simulink model "sampleModel20"  (R2021a)
settings: Solver=VariableStepAuto  StartTime=0.0  StopTime=10.0  RelTol=1e-3
undefined symbols (not defined in the file): DiscIntNeverNeededParam, magnitude, Newton, Raphson
libraries: simulink x274, pid_lib x17
(part 2 of 16)

== system sampleModel20/cfblk77/cfblk9 ==
  cfblk1 : Inport
  cfblk8 : Inport  Port=2
  cfblk9 : Inport  Port=3
  cfblk10 : Inport  Port=4
  cfblk11 : Inport  Port=5
  cfblk{12..17} (6 alike) : Delay  SampleTime=1
  cfblk3 : Sin  TimeSource=Use external signal  SampleTime=0
  cfblk4 : Assignment  DiagnosticForDimensions=Warning  IndexOptions=Index vector (dialog)  Indices=1  OutputSizes=1
  cfblk5 : Subsystem
  cfblk6 : Subsystem
  cfblk7 : Subsystem
  cfblk2 : Outport
  wires:
  cfblk1/1 -> cfblk5/1(cfblk1)
  cfblk6/1(cfblk2) -> cfblk7/1(cfblk1)
  cfblk8/1 -> cfblk4/1
  cfblk9/1 -> cfblk4/2
  cfblk5/1(cfblk2) -> cfblk3/1
  cfblk11/1 -> cfblk2/1, cfblk7/4(cfblk6)
  cfblk10/1 -> cfblk5/3(cfblk8)
  cfblk4/1 -> cfblk7/2(cfblk4)
  cfblk5/2(cfblk12) -> cfblk6/2(cfblk12)
  cfblk7/2(cfblk7) -> cfblk14/1, cfblk15/1, cfblk16/1
  cfblk6/3(cfblk15) -> cfblk7/3(cfblk5)
  cfblk3/1 -> cfblk12/1
  cfblk12/1 -> cfblk5/4(cfblk9)
  cfblk7/1(cfblk2) -> cfblk13/1
  cfblk13/1 -> cfblk6/1(cfblk1)
  cfblk14/1 -> cfblk6/3(cfblk13)
  cfblk15/1 -> cfblk5/5(cfblk10)
  cfblk16/1 -> cfblk5/6(cfblk11)
  cfblk6/2(cfblk14) -> cfblk17/1
  cfblk17/1 -> cfblk5/2(cfblk7)

== system sampleModel20/cfblk78/cfblk10 ==
  cfblk1 : Inport
  cfblk9 : Inport  Port=2
  cfblk10 : Inport  Port=3
  cfblk11 : Inport  Port=4
  cfblk12 : Inport  Port=5
  cfblk{14..17} (4 alike) : Delay  SampleTime=1
  cfblk3 : pid_lib/PID Controller (2DOF)  Controller=PID  Form=Parallel  TimeDomain=Discrete-time  UseExternalTs=off  SampleTime=1  IntegratorMethod=Forward Euler  FilterMethod=Forward Euler  ControllerParametersSource=internal  P=1  I=1  D=0  UseFilter=on  N=100  b=1  c=1  TunerSelectOption=Transfer Function Based (PID Tuner App)  InitialConditionSource=internal  InitialConditionForIntegrator=0  InitialConditionForFilter=0  DifferentiatorICPrevScaledInput=0  ExternalReset=none  TrackingMode=off  Kt=1  LimitOutput=off  SatLimitsSource=internal  UpperSaturationLimit=inf  LowerSaturationLimit=-inf  LinearizeAsGain=off  AntiWindupMode=none  Kb=1  POutMin=[]  POutMax=[]  IOutMin=[]  IOutMax=[]  DOutMin=[]  DOutMax=[]  NOutMin=[]  NOutMax=[]  bOutMin=[]  bOutMax=[]  cOutMin=[]  cOutMax=[]  SumOutMin=[]  SumOutMax=[]  SaturationOutMin=[]  SaturationOutMax=[]  PParamMin=[]  PParamMax=[]  IParamMin=[]  IParamMax=[]  DParamMin=[]  DParamMax=[]  NParamMin=[]  NParamMax=[]  bParamMin=[]  bParamMax=[]  cParamMin=[]  cParamMax=[]  KbParamMin=[]  KbParamMax=[]  KtParamMin=[]  KtParamMax=[]  KbOutMin=[]  KbOutMax=[]  KtOutMin=[]  KtOutMax=[]  IntegratorOutMin=[]  IntegratorOutMax=[]  FilterOutMin=[]  FilterOutMax=[]  SumI1OutMin=[]  SumI1OutMax=[]  SumI2OutMin=[]  SumI2OutMax=[]  SumI3OutMin=[]  SumI3OutMax=[]  SumI4OutMin=[]  SumI4OutMax=[]  SumDOutMin=[]  SumDOutMax=[]  Sum1OutMin=[]  Sum1OutMax=[]  Sum2OutMin=[]  Sum2OutMax=[]  Sum3OutMin=[]  Sum3OutMax=[]  DifferentiatorOutMin=[]  DifferentiatorOutMax=[]  FilterDiffOutCoefMin=[]  FilterDiffOutCoefMax=[]  ReciprocalOutMin=[]  ReciprocalOutMax=[]  SumDenOutMin=[]  SumDenOutMax=[]  SumNumOutMin=[]  SumNumOutMax=[]  DivideOutMin=[]  DivideOutMax=[]  UdiffTsProdOutMin=[]  UdiffTsProdOutMax=[]  NTsProdOutMin=[]  NTsProdOutMax=[]  UintegralTsProdOutMin=[]  UintegralTsProdOutMax=[]  UngainTsProdOutMin=[]  UngainTsProdOutMax=[]  IntegratorContinuousStateAttributes=''  IntegratorStateMustResolveToSignalObject=off  IntegratorRTWStateStorageClass=Auto  FilterContinuousStateAttributes=''  FilterStateMustResolveToSignalObject=off  FilterRTWStateStorageClass=Auto  ParallelPVariant=InternalParameters  IdealPVariant=Disabled  IVariant=InternalParameters  DVariant=InternalParameters  bVariant=InternalParameters  cVariant=InternalParameters  IntegratorVariant=Discrete  SatVariant=Disabled  AWVariant=Passthrough  PCopyVariant=Disabled  TRVariant=Disabled  FdbkBlocksVariant=Forward  IdealPFdbkVariant=Disabled  SatFdbkVariant=Disabled  DerivativeFilterVariant=ForwardEulerFilter  NVariant=InternalParameters  NCopyVariant=Disabled  FilterICVariant=InternalICsFilter  IntegratorICVariant=InternalICs  ExternalResetVariant=Disabled  TRSumVariant=Passthrough  SumFdbkVariant=Disabled  SumVariant=Sum_PID  TsampFilterVariant=InternalTs  TsampNgainVariant=Passthrough  TsampIntegralVariant=Passthrough  ExternalSaturationOutDataTypeStr=Inherit: Same as second input
      settings: SourceProductBaseCode=SL
  cfblk4 : Sum  Inputs=+
  cfblk5 : Sum  Inputs=--
  cfblk6 : Subsystem
  cfblk7 : Subsystem
  cfblk8 : Subsystem
  cfblk2 : Outport
  cfblk13 : Outport  Port=2
  wires:
  cfblk1/1 -> cfblk2/1, cfblk8/5(cfblk7)
  cfblk8/1(cfblk2) -> cfblk7/2(cfblk9)
  cfblk11/1 -> cfblk8/1(cfblk1)
  cfblk4/1 -> cfblk5/1
  cfblk6/2(cfblk7) -> cfblk4/1
  cfblk9/1 -> cfblk7/3(cfblk10)
  cfblk12/1 -> cfblk3/1
  cfblk7/1(cfblk2) -> cfblk6/1(cfblk1)
  cfblk10/1 -> cfblk8/2(cfblk4)
  cfblk8/2(cfblk8) -> cfblk5/2
  cfblk6/3(cfblk8) -> cfblk3/2
  cfblk8/3(cfblk9) -> cfblk13/1
  cfblk6/1(cfblk2) -> cfblk14/1
  cfblk14/1 -> cfblk7/1(cfblk1)
  cfblk5/1 -> cfblk15/1
  cfblk15/1 -> cfblk8/3(cfblk5)
  cfblk3/1 -> cfblk16/1
  cfblk16/1 -> cfblk7/4(cfblk11)
  cfblk7/2(cfblk12) -> cfblk17/1
  cfblk17/1 -> cfblk8/4(cfblk6)

== system sampleModel20/cfblk78/cfblk7 ==
  cfblk1 : Inport
  cfblk8 : Inport  Port=2
  cfblk9 : Inport  Port=3
  cfblk10 : Inport  Port=4
  cfblk11 : Inport  Port=5
  cfblk12 : Inport  Port=6
  cfblk13 : Delay  SampleTime=1
  cfblk14 : Delay  SampleTime=1
  cfblk15 : Delay  SampleTime=1
  cfblk3 : DiscreteFir  SampleTime=1
  cfblk4 : ComplexToRealImag
  cfblk5 : ComplexToRealImag
  cfblk6 : Subsystem
  cfblk7 : Subsystem
  cfblk2 : Outport
  wires:
  cfblk4/1 -> cfblk3/1
  cfblk8/1 -> cfblk4/1
  cfblk4/2 -> cfblk5/1
  cfblk9/1 -> cfblk6/1(cfblk1)
  cfblk3/1 -> cfblk2/1
  cfblk1/1 -> cfblk7/2(cfblk8)
  cfblk10/1 -> cfblk6/2(cfblk9)
  cfblk11/1 -> cfblk7/3(cfblk9)
  cfblk12/1 -> cfblk6/3(cfblk10)
  cfblk7/1(cfblk2) -> cfblk6/4(cfblk11)
  cfblk6/1(cfblk2) -> cfblk13/1
  cfblk13/1 -> cfblk7/1(cfblk1)
  cfblk6/2(cfblk12) -> cfblk14/1
  cfblk14/1 -> cfblk7/4(cfblk10)
  cfblk6/3(cfblk13) -> cfblk15/1
  cfblk15/1 -> cfblk7/5(cfblk11)

== system sampleModel20/cfblk78/cfblk8 ==
  cfblk1 : Inport
  cfblk7 : Inport  Port=2
  cfblk8 : Inport  Port=3
  cfblk9 : Inport  Port=4
  cfblk10 : Inport  Port=5
  cfblk{11..14} (4 alike) : Delay  SampleTime=1
  cfblk3 : Sqrt  SaturateOnIntegerOverflow=on
  cfblk4 : Sum  Inputs=+-
  cfblk5 : Subsystem
  cfblk6 : Subsystem
  cfblk2 : Outport
  wires:
  cfblk6/1(cfblk2) -> cfblk3/1
  cfblk5/1(cfblk2) -> cfblk6/1(cfblk1)
  cfblk6/2(cfblk15) -> cfblk4/1
  cfblk1/1 -> cfblk5/1(cfblk1), cfblk6/7(cfblk13)
  cfblk8/1 -> cfblk4/2
  cfblk10/1 -> cfblk6/2(cfblk8), cfblk6/8(cfblk14)
  cfblk7/1 -> cfblk2/1, cfblk6/5(cfblk11)
  cfblk3/1 -> cfblk11/1, cfblk12/1
  cfblk9/1 -> cfblk5/2(cfblk14)
  cfblk4/1 -> cfblk13/1, cfblk14/1
  cfblk5/2(cfblk17) -> cfblk6/4(cfblk10)
  cfblk11/1 -> cfblk6/3(cfblk9)
  cfblk12/1 -> cfblk6/6(cfblk12)
  cfblk13/1 -> cfblk5/3(cfblk15)
  cfblk14/1 -> cfblk5/4(cfblk16)

== system sampleModel20/cfblk78/cfblk9 ==
  cfblk1 : Inport
  cfblk10 : Subsystem
  cfblk11 : Subsystem
  cfblk12 : Subsystem
  cfblk{14..18} (5 alike) : Delay  SampleTime=1
  cfblk3 : PermuteDimensions
  cfblk4 : PermuteDimensions
  cfblk5 : Product  Inputs=*
  cfblk6 : DotProduct  InputSameDT=on  OutDataTypeStr=Inherit: Inherit via internal rule
  cfblk7 : Signum
  cfblk8 : simulink/Math Operations/MinMax Running Resettable  Function=min  vinit=0.0
  cfblk9 : Sum  Inputs=|++
  cfblk2 : Outport
  cfblk13 : Outport  Port=2
  wires:
  cfblk8/1 -> cfblk5/1, cfblk12/7(cfblk13)
  cfblk7/1 -> cfblk12/3(cfblk9), cfblk12/4(cfblk10), cfblk15/1
  cfblk3/1 -> cfblk12/2(cfblk8), cfblk18/1
  cfblk1/1 -> cfblk6/2, cfblk10/3(cfblk11)
  cfblk4/1 -> cfblk7/1, cfblk12/1(cfblk1), cfblk17/1
  cfblk6/1 -> cfblk8/2
  cfblk11/2(cfblk8) -> cfblk2/1, cfblk10/2(cfblk10), cfblk12/5(cfblk11), cfblk12/6(cfblk12)
  cfblk10/1(cfblk2) -> cfblk13/1
  cfblk10/2(cfblk12) -> cfblk4/1
  cfblk5/1 -> cfblk9/2, cfblk3/1
  cfblk9/1 -> cfblk11/1(cfblk1)
  cfblk11/1(cfblk2) -> cfblk14/1
  cfblk14/1 -> cfblk9/1
  cfblk15/1 -> cfblk8/1
  cfblk12/1(cfblk2) -> cfblk16/1
  cfblk16/1 -> cfblk10/1(cfblk1)
  cfblk17/1 -> cfblk11/2(cfblk7)
  cfblk18/1 -> cfblk6/1

== system sampleModel20/cfblk79/cfblk8 ==
  cfblk1 : Inport
  cfblk6 : Inport  Port=2
  cfblk7 : Inport  Port=3
  cfblk3 : Gain  Gain=[911882723.754040]
  cfblk4 : Gain  Gain=[-751288101.228312]
  cfblk5 : Product  Inputs=**
  cfblk9 : Delay  SampleTime=1
  cfblk2 : Outport
  cfblk8 : Outport  Port=2
  wires:
  cfblk1/1 -> cfblk3/1
  cfblk5/1 -> cfblk4/1
  cfblk7/1 -> cfblk2/1
  cfblk6/1 -> cfblk8/1
  cfblk3/1 -> cfblk5/2
  cfblk4/1 -> cfblk9/1
  cfblk9/1 -> cfblk5/1

== system sampleModel20/cfblk79/cfblk9 ==
  cfblk1 : Inport
  cfblk9 : Inport  Port=2
  cfblk10 : Inport  Port=3
  cfblk11 : Inport  Port=4
  cfblk12 : Delay  SampleTime=1
  cfblk13 : Delay  SampleTime=1
  cfblk3 : Signum
  cfblk4 : Rounding
  cfblk5 : Sin  TimeSource=Use external signal  SampleTime=0
  cfblk6 : Sqrt  Operator=rSqrt  AlgorithmType=Newton-Raphson  SaturateOnIntegerOverflow=on
  cfblk7 : Subsystem
  cfblk8 : Subsystem
  cfblk2 : Outport
  wires:
  cfblk7/1(cfblk2) -> cfblk8/1(cfblk1)
  cfblk1/1 -> cfblk3/1
  cfblk4/1 -> cfblk6/1
  cfblk8/2(cfblk8) -> cfblk5/1
  cfblk9/1 -> cfblk4/1
  cfblk7/2(cfblk14) -> cfblk8/2(cfblk6)
  cfblk10/1 -> cfblk2/1
  cfblk3/1 -> cfblk7/2(cfblk11)
  cfblk6/1 -> cfblk7/3(cfblk12)
  cfblk11/1 -> cfblk7/4(cfblk13)
  cfblk8/1(cfblk2) -> cfblk12/1
  cfblk12/1 -> cfblk7/1(cfblk1)
  cfblk5/1 -> cfblk13/1
  cfblk13/1 -> cfblk8/3(cfblk7)

== system sampleModel20/cfblk80/cfblk6 ==
  cfblk1 : Inport
  cfblk9 : Inport  Port=2
  cfblk10 : Inport  Port=3
  cfblk11 : Inport  Port=4
  cfblk12 : Inport  Port=5
  cfblk14 : Delay  SampleTime=1
  cfblk15 : Delay  SampleTime=1
  cfblk16 : Delay  SampleTime=1
  cfblk3 : Sum  Inputs=+-
  cfblk4 : Gain  Gain=[17475078.274837]
  cfblk5 : DotProduct  InputSameDT=on  OutDataTypeStr=Inherit: Inherit via internal rule
  cfblk6 : Subsystem
  cfblk7 : Subsystem
  cfblk8 : Subsystem
  cfblk2 : Outport
  cfblk13 : Outport  Port=2
  wires:
  cfblk12/1 -> cfblk7/1(cfblk1), cfblk6/2(cfblk6), cfblk6/4(cfblk8)
  cfblk9/1 -> cfblk8/1(cfblk1)
  cfblk6/1(cfblk2) -> cfblk7/2(cfblk9)
  cfblk4/1 -> cfblk3/1, cfblk8/4(cfblk15), cfblk8/5(cfblk16)
  cfblk3/1 -> cfblk13/1
  cfblk1/1 -> cfblk2/1
  cfblk8/1(cfblk2) -> cfblk6/1(cfblk1), cfblk16/1
  cfblk10/1 -> cfblk5/1, cfblk6/3(cfblk7)
  cfblk11/1 -> cfblk3/2
  cfblk7/1(cfblk2) -> cfblk5/2, cfblk14/1
  cfblk14/1 -> cfblk8/3(cfblk14)
  cfblk5/1 -> cfblk15/1
  cfblk15/1 -> cfblk8/2(cfblk13)
  cfblk16/1 -> cfblk4/1

== system sampleModel20/cfblk81/cfblk4 ==
  cfblk1 : Inport
  cfblk13 : Inport  Port=2
  cfblk14 : Inport  Port=3
  cfblk15 : Inport  Port=4
  cfblk16 : Inport  Port=5
  cfblk10 : Subsystem
  cfblk11 : Subsystem
  cfblk12 : Subsystem
  cfblk{17..21} (5 alike) : Delay  SampleTime=1
  cfblk3 : pid_lib/PID Controller  Controller=PID  Form=Parallel  TimeDomain=Discrete-time  UseExternalTs=off  SampleTime=1  IntegratorMethod=Forward Euler  FilterMethod=Forward Euler  ControllerParametersSource=internal  P=1  I=1  D=0  UseFilter=on  N=100  TunerSelectOption=Transfer Function Based (PID Tuner App)  InitialConditionSource=internal  InitialConditionForIntegrator=0  InitialConditionForFilter=0  DifferentiatorICPrevScaledInput=0  ExternalReset=none  TrackingMode=off  Kt=1  LimitOutput=off  SatLimitsSource=internal  UpperSaturationLimit=inf  LowerSaturationLimit=-inf  LinearizeAsGain=off  AntiWindupMode=none  Kb=1  POutMin=[]  POutMax=[]  IOutMin=[]  IOutMax=[]  DOutMin=[]  DOutMax=[]  NOutMin=[]  NOutMax=[]  SumOutMin=[]  SumOutMax=[]  SaturationOutMin=[]  SaturationOutMax=[]  PParamMin=[]  PParamMax=[]  IParamMin=[]  IParamMax=[]  DParamMin=[]  DParamMax=[]  NParamMin=[]  NParamMax=[]  KbParamMin=[]  KbParamMax=[]  KtParamMin=[]  KtParamMax=[]  KbOutMin=[]  KbOutMax=[]  KtOutMin=[]  KtOutMax=[]  IntegratorOutMin=[]  IntegratorOutMax=[]  FilterOutMin=[]  FilterOutMax=[]  SumI1OutMin=[]  SumI1OutMax=[]  SumI2OutMin=[]  SumI2OutMax=[]  SumI3OutMin=[]  SumI3OutMax=[]  SumI4OutMin=[]  SumI4OutMax=[]  SumDOutMin=[]  SumDOutMax=[]  DifferentiatorOutMin=[]  DifferentiatorOutMax=[]  FilterDiffOutCoefMin=[]  FilterDiffOutCoefMax=[]  ReciprocalOutMin=[]  ReciprocalOutMax=[]  SumDenOutMin=[]  SumDenOutMax=[]  SumNumOutMin=[]  SumNumOutMax=[]  DivideOutMin=[]  DivideOutMax=[]  UdiffTsProdOutMin=[]  UdiffTsProdOutMax=[]  NTsProdOutMin=[]  NTsProdOutMax=[]  UintegralTsProdOutMin=[]  UintegralTsProdOutMax=[]  UngainTsProdOutMin=[]  UngainTsProdOutMax=[]  IntegratorContinuousStateAttributes=''  IntegratorStateMustResolveToSignalObject=off  IntegratorRTWStateStorageClass=Auto  FilterContinuousStateAttributes=''  FilterStateMustResolveToSignalObject=off  FilterRTWStateStorageClass=Auto  ParallelPVariant=InternalParameters  IdealPVariant=Disabled  IVariant=InternalParameters  DVariant=InternalParameters  IntegratorVariant=Discrete  SatVariant=Disabled  AWVariant=Passthrough  PCopyVariant=Disabled  TRVariant=Disabled  FdbkBlocksVariant=Forward  IdealPFdbkVariant=Disabled  SatFdbkVariant=Disabled  DerivativeFilterVariant=ForwardEulerFilter  NVariant=InternalParameters  NCopyVariant=Disabled  FilterICVariant=InternalICsFilter  IntegratorICVariant=InternalICs  ExternalResetVariant=Disabled  TRSumVariant=Passthrough  SumFdbkVariant=Disabled  SumVariant=Sum_PID  TsampFilterVariant=InternalTs  TsampNgainVariant=Passthrough  TsampIntegralVariant=Passthrough  ExternalSaturationOutDataTypeStr=Inherit: Same as second input
  cfblk4 : DotProduct  InputSameDT=on  OutDataTypeStr=Inherit: Inherit via internal rule
  cfblk5 : Signum
  cfblk6 : Rounding
  cfblk7 : Sqrt  SaturateOnIntegerOverflow=on
  cfblk8 : Reshape
  cfblk9 : MinMax  Function=max  Inputs=2
  cfblk2 : Outport
  wires:
  cfblk9/1 -> cfblk12/1(cfblk1)
  cfblk10/1(cfblk2) -> cfblk3/1, cfblk4/2
  cfblk3/1 -> cfblk12/2(cfblk9), cfblk12/7(cfblk14)
  cfblk15/1 -> cfblk12/3(cfblk10), cfblk12/6(cfblk13)
  cfblk6/1 -> cfblk9/1
  cfblk7/1 -> cfblk5/1
  cfblk12/1(cfblk2) -> cfblk11/3(cfblk9), cfblk11/4(cfblk10), cfblk17/1
  cfblk4/1 -> cfblk20/1, cfblk21/1
  cfblk13/1 -> cfblk11/1(cfblk1)
  cfblk14/1 -> cfblk6/1
  cfblk11/1(cfblk2) -> cfblk7/1
  cfblk8/1 -> cfblk9/2
  cfblk1/1 -> cfblk10/3(cfblk9)
  cfblk11/2(cfblk11) -> cfblk2/1
  cfblk16/1 -> cfblk8/1
  cfblk11/3(cfblk12) -> cfblk4/1, cfblk19/1
  cfblk17/1 -> cfblk10/1(cfblk1)
  cfblk5/1 -> cfblk18/1
  cfblk18/1 -> cfblk10/2(cfblk8)
  cfblk19/1 -> cfblk12/5(cfblk12)
  cfblk20/1 -> cfblk12/4(cfblk11)
  cfblk21/1 -> cfblk11/2(cfblk8)

== system sampleModel20/cfblk81/cfblk5 ==
  cfblk1 : Inport
  cfblk5 : Inport  Port=2
  cfblk6 : Inport  Port=3
  cfblk7 : Inport  Port=4
  cfblk3 : simulink/Math Operations/Slider Gain  gain=1  low=0  high=2
  cfblk4 : Subsystem
  cfblk2 : Outport
  cfblk8 : Outport  Port=2
  wires:
  cfblk3/1 -> cfblk8/1
  cfblk4/1(cfblk2) -> cfblk2/1
  cfblk1/1 -> cfblk4/1(cfblk1)
  cfblk7/1 -> cfblk4/2(cfblk6)
  cfblk4/2(cfblk7) -> cfblk3/1

== system sampleModel20/cfblk81/cfblk6 ==
  cfblk1 : Inport
  cfblk8 : Inport  Port=2
  cfblk9 : Inport  Port=3
  cfblk10 : Inport  Port=4
  cfblk11 : Inport  Port=5
  cfblk12 : Delay  SampleTime=1
  cfblk3 : DiscreteFir  SampleTime=1
  cfblk4 : ComplexToRealImag
  cfblk5 : Sum  Inputs=|++
  cfblk6 : Sum  Inputs=|++
  cfblk7 : Subsystem
  cfblk2 : Outport
  wires:
  cfblk1/1 -> cfblk3/1
  cfblk4/1 -> cfblk6/2
  cfblk6/1 -> cfblk5/1
  cfblk11/1 -> cfblk4/1
  cfblk3/1 -> cfblk2/1
  cfblk9/1 -> cfblk5/2
  cfblk8/1 -> cfblk7/1(cfblk1)
  cfblk10/1 -> cfblk7/2(cfblk10), cfblk7/4(cfblk12)
  cfblk4/2 -> cfblk7/3(cfblk11), cfblk7/5(cfblk13), cfblk7/6(cfblk14)
  cfblk5/1 -> cfblk12/1
  cfblk12/1 -> cfblk6/1

== system sampleModel20/cfblk81/cfblk7 ==
  cfblk1 : Inport
  cfblk10 : Inport  Port=2
  cfblk11 : Inport  Port=3
  cfblk12 : Inport  Port=4
  cfblk13 : Inport  Port=5
  cfblk16 : Delay  SampleTime=1
  cfblk17 : Delay  SampleTime=1
  cfblk18 : Delay  SampleTime=1
  cfblk3 : DiscreteIntegrator  ICPrevOutput=DiscIntNeverNeededParam  ICPrevScaledInput=DiscIntNeverNeededParam
  cfblk4 : Product  Inputs=*
  cfblk5 : MinMax  Function=max  Inputs=2
  cfblk6 : ComplexToRealImag
  cfblk7 : Product  Inputs=*
  cfblk8 : Sin  TimeSource=Use external signal  SampleTime=0
  cfblk9 : Subsystem
  cfblk2 : Outport
  cfblk14 : Outport  Port=2
  cfblk15 : Outport  Port=3
  wires:
  cfblk8/1 -> cfblk2/1, cfblk9/6(cfblk15)
  cfblk7/1 -> cfblk14/1
  cfblk10/1 -> cfblk15/1
  cfblk4/1 -> cfblk5/1
  cfblk1/1 -> cfblk9/1(cfblk1), cfblk9/5(cfblk14)
  cfblk12/1 -> cfblk8/1
  cfblk3/1 -> cfblk6/1
  cfblk13/1 -> cfblk7/1
  cfblk5/1 -> cfblk16/1, cfblk17/1
  cfblk9/1(cfblk2) -> cfblk4/1
  cfblk11/1 -> cfblk9/3(cfblk12)
  cfblk9/2(cfblk17) -> cfblk5/2
  cfblk6/2 -> cfblk9/4(cfblk13)
  cfblk16/1 -> cfblk9/2(cfblk11)
  cfblk17/1 -> cfblk9/7(cfblk16)
  cfblk6/1 -> cfblk18/1
  cfblk18/1 -> cfblk3/1

== system sampleModel20/cfblk82/cfblk4 ==
  cfblk1 : Inport
  cfblk13 : Inport  Port=2
  cfblk14 : Inport  Port=3
  cfblk15 : Inport  Port=4
  cfblk10 : Subsystem
  cfblk11 : Subsystem
  cfblk12 : Subsystem
  cfblk{18..21} (4 alike) : Delay  SampleTime=1
  cfblk3 : ComplexToMagnitudeAngle
  cfblk4 : ComplexToMagnitudeAngle
  cfblk5 : Rounding
  cfblk6 : Signum
  cfblk7 : Polyval  Coefs=[ +2.081618890e-019, -1.441693666e-014, +4.719686976e-010, -8.536869453e-006, +1.621573104e-001, -8.087801117e+001 ]
  cfblk8 : Subsystem
  cfblk9 : Subsystem
  cfblk2 : Outport
  cfblk16 : Outport  Port=2
  cfblk17 : Outport  Port=3
  wires:
  cfblk13/1 -> cfblk17/1
  cfblk9/1(cfblk2) -> cfblk16/1
  cfblk14/1 -> cfblk4/1
  cfblk4/1 -> cfblk7/1
  cfblk5/1 -> cfblk12/1(cfblk1), cfblk9/3(cfblk10), cfblk11/4(cfblk13)
  cfblk15/1 -> cfblk3/1
  cfblk11/2(cfblk15) -> cfblk6/1
  cfblk1/1 -> cfblk5/1, cfblk11/5(cfblk14)
  cfblk7/1 -> cfblk2/1
  cfblk12/1(cfblk2) -> cfblk10/1(cfblk1)
  cfblk10/1(cfblk2) -> cfblk8/2(cfblk7)
  cfblk3/1 -> cfblk9/1(cfblk1)
  cfblk3/2 -> cfblk12/2(cfblk11), cfblk10/4(cfblk13)
  cfblk6/1 -> cfblk9/6(cfblk13), cfblk19/1
  cfblk4/2 -> cfblk8/3(cfblk8), cfblk12/4(cfblk13), cfblk9/5(cfblk12)
  cfblk10/2(cfblk14) -> cfblk9/2(cfblk9)
  cfblk8/1(cfblk2) -> cfblk11/1(cfblk1)
  cfblk8/3(cfblk11) -> cfblk11/2(cfblk11), cfblk21/1
  cfblk10/3(cfblk15) -> cfblk8/4(cfblk9), cfblk11/3(cfblk12), cfblk9/4(cfblk11)
  cfblk11/1(cfblk2) -> cfblk18/1
  cfblk18/1 -> cfblk8/1(cfblk1)
  cfblk19/1 -> cfblk10/2(cfblk11)
  cfblk8/2(cfblk10) -> cfblk20/1
  cfblk20/1 -> cfblk10/3(cfblk12)
  cfblk21/1 -> cfblk12/3(cfblk12)

== system sampleModel20/cfblk83/cfblk4 ==
  cfblk1 : Inport
  cfblk9 : Inport  Port=2
  cfblk10 : Inport  Port=3
  cfblk11 : Inport  Port=4
  cfblk12 : Inport  Port=5
  cfblk3 : DotProduct  InputSameDT=on  OutDataTypeStr=Inherit: Inherit via internal rule
  cfblk4 : simulink/Math Operations/MinMax Running Resettable  Function=min  vinit=0.0
  cfblk5 : simulink/Math Operations/Slider Gain  gain=1  low=0  high=2
  cfblk6 : Polyval  Coefs=[ +2.081618890e-019, -1.441693666e-014, +4.719686976e-010, -8.536869453e-006, +1.621573104e-001, -8.087801117e+001 ]
  cfblk7 : MinMax  Function=max  Inputs=3
  cfblk8 : Squeeze
  cfblk2 : Outport
  cfblk13 : Outport  Port=2
  wires:
  cfblk6/1 -> cfblk7/1
  cfblk1/1 -> cfblk13/1
  cfblk3/1 -> cfblk2/1
  cfblk7/1 -> cfblk3/1
  cfblk12/1 -> cfblk3/2
  cfblk10/1 -> cfblk8/1
  cfblk9/1 -> cfblk6/1
  cfblk4/1 -> cfblk7/2
  cfblk11/1 -> cfblk7/3
  cfblk5/1 -> cfblk4/1
  cfblk8/1 -> cfblk4/2, cfblk5/1

== system sampleModel20/cfblk83/cfblk5 ==
  cfblk1 : Inport
  cfblk7 : Inport  Port=2
  cfblk8 : Inport  Port=3
  cfblk12 : Delay  SampleTime=1
  cfblk3 : Sum  Inputs=+
  cfblk4 : Subsystem
  cfblk5 : Subsystem
  cfblk6 : Subsystem
  cfblk2 : Outport
  cfblk9 : Outport  Port=2
  cfblk10 : Outport  Port=3
  cfblk11 : Outport  Port=4
  wires:
  cfblk7/1 -> cfblk6/1(cfblk1)
  cfblk6/1(cfblk2) -> cfblk5/1(cfblk1)
  cfblk4/1(cfblk2) -> cfblk3/1
  cfblk5/1(cfblk2) -> cfblk10/1
  cfblk6/2(cfblk7) -> cfblk2/1
  cfblk1/1 -> cfblk11/1, cfblk5/3(cfblk10)
  cfblk8/1 -> cfblk4/2(cfblk9)
  cfblk3/1 -> cfblk9/1, cfblk5/2(cfblk9)
  cfblk4/2(cfblk10) -> cfblk6/2(cfblk6)
  cfblk6/3(cfblk8) -> cfblk12/1
  cfblk12/1 -> cfblk4/1(cfblk1)

== system sampleModel20/cfblk83/cfblk6 ==
  cfblk1 : Inport
  cfblk6 : Inport  Port=2
  cfblk3 : DiscreteTransferFcn  SampleTime=1
  cfblk4 : Polyval  Coefs=[ +2.081618890e-019, -1.441693666e-014, +4.719686976e-010, -8.536869453e-006, +1.621573104e-001, -8.087801117e+001 ]
  cfblk5 : Subsystem
  cfblk2 : Outport
  cfblk7 : Outport  Port=2
  wires:
  cfblk3/1 -> cfblk7/1
  cfblk6/1 -> cfblk3/1, cfblk5/1(cfblk1)
  cfblk1/1 -> cfblk4/1
  cfblk4/1 -> cfblk2/1, cfblk5/2(cfblk9)

== system sampleModel20/cfblk83/cfblk7 ==
  cfblk1 : Inport
  cfblk12 : Inport  Port=2
  cfblk13 : Inport  Port=3
  cfblk14 : Inport  Port=4
  cfblk15 : Inport  Port=5
  cfblk16 : Inport  Port=6
  cfblk17 : Inport  Port=7
  cfblk10 : Subsystem
  cfblk11 : Subsystem
  cfblk{18..21} (4 alike) : Delay  SampleTime=1
  cfblk3 : Delay  ShowEnablePort=on  SampleTime=1
      settings: InputPortMap=u0,e6
  cfblk4 : Product  Inputs=*
  cfblk5 : Sum  Inputs=-+
  cfblk6 : ComplexToRealImag
  cfblk7 : Subsystem
  cfblk8 : Subsystem
  cfblk9 : Subsystem
  cfblk2 : Outport
  wires:
  cfblk17/1 -> cfblk6/1, cfblk11/4(cfblk7)
  cfblk15/1 -> cfblk5/1
  cfblk11/1(cfblk2) -> cfblk20/1, cfblk21/1
  cfblk9/1(cfblk2) -> cfblk5/2
  cfblk16/1 -> cfblk10/2(cfblk7), cfblk11/2(cfblk5)
  cfblk12/1 -> cfblk7/1(cfblk1)
  cfblk8/1(cfblk2) -> cfblk2/1
  cfblk14/1 -> cfblk7/2(cfblk12), cfblk11/1(cfblk1)
  cfblk5/1 -> cfblk10/3(cfblk8)
  cfblk10/1(cfblk2) -> cfblk7/3(cfblk13), cfblk11/3(cfblk6)
  cfblk3/1 -> cfblk11/6(cfblk9), cfblk19/1
  cfblk1/1 -> cfblk9/2(cfblk6)
  cfblk9/2(cfblk9) -> cfblk7/4(cfblk14), cfblk8/2(cfblk7)
  cfblk7/1(cfblk2) -> cfblk8/3(cfblk8), cfblk18/1
  cfblk4/1 -> cfblk7/5(cfblk15), cfblk11/5(cfblk8)
  cfblk6/1 -> cfblk8/1(cfblk1)
  cfblk13/1 -> cfblk7/6(cfblk16), cfblk9/4(cfblk8)
  cfblk6/2 -> cfblk4/1
  cfblk8/2(cfblk10) -> cfblk3/1, cfblk3/2
  cfblk18/1 -> cfblk9/3(cfblk7)
  cfblk19/1 -> cfblk9/1(cfblk1)
  cfblk20/1 -> cfblk10/1(cfblk1)
  cfblk21/1 -> cfblk8/4(cfblk9)

== system sampleModel20/cfblk84/cfblk10 ==
  cfblk1 : Inport
  cfblk12 : Inport  Port=2
  cfblk13 : Inport  Port=3
  cfblk14 : Inport  Port=4
  cfblk15 : Inport  Port=5
  cfblk16 : Inport  Port=6
  cfblk17 : Inport  Port=7
  cfblk10 : Subsystem
  cfblk11 : Subsystem
  cfblk18 : Delay  SampleTime=1
  cfblk19 : Delay  SampleTime=1
  cfblk20 : Delay  SampleTime=1
  cfblk3 : Product
  cfblk4 : Sqrt  SaturateOnIntegerOverflow=on
  cfblk5 : Product  Inputs=*
  cfblk6 : DotProduct  InputSameDT=on  OutDataTypeStr=Inherit: Inherit via internal rule
  cfblk7 : Sin  TimeSource=Use external signal  SampleTime=0
  cfblk8 : ComplexToRealImag
  cfblk9 : Subsystem
  cfblk2 : Outport
  wires:
  cfblk4/1 -> cfblk3/1
  cfblk12/1 -> cfblk3/2
  cfblk15/1 -> cfblk6/1
  cfblk1/1 -> cfblk7/1
  cfblk17/1 -> cfblk5/1
  cfblk10/1(cfblk2) -> cfblk4/1
  cfblk5/1 -> cfblk11/2(cfblk10)
  cfblk7/1 -> cfblk11/3(cfblk11)
  cfblk6/1 -> cfblk9/1(cfblk1)
  cfblk10/2(cfblk13) -> cfblk8/1
  cfblk14/1 -> cfblk11/4(cfblk12)
  cfblk13/1 -> cfblk2/1
  cfblk16/1 -> cfblk6/2
  cfblk11/1(cfblk2) -> cfblk10/3(cfblk12)
  cfblk10/3(cfblk14) -> cfblk9/2(cfblk9)
  cfblk8/2 -> cfblk9/3(cfblk10)
  cfblk3/1 -> cfblk18/1
  cfblk18/1 -> cfblk11/1(cfblk1)
  cfblk8/1 -> cfblk19/1
  cfblk19/1 -> cfblk10/1(cfblk1)
  cfblk9/1(cfblk2) -> cfblk20/1
  cfblk20/1 -> cfblk10/2(cfblk11)

== system sampleModel20/cfblk84/cfblk5 ==
  cfblk1 : Inport
  cfblk10 : Inport  Port=2
  cfblk11 : Inport  Port=3
  cfblk12 : Inport  Port=4
  cfblk{14..19} (6 alike) : Delay  SampleTime=1
  cfblk3 : Abs
  cfblk4 : Rounding
  cfblk5 : Sum  Inputs=+-
  cfblk6 : Subsystem
  cfblk7 : Subsystem
  cfblk8 : Subsystem
  cfblk9 : Subsystem
  cfblk2 : Outport
  cfblk13 : Outport  Port=2
  wires:
  cfblk8/1(cfblk2) -> cfblk6/1(cfblk1)
  cfblk10/1 -> cfblk2/1
  cfblk4/1 -> cfblk7/1(cfblk1)
  cfblk3/1 -> cfblk16/1, cfblk17/1
  cfblk9/1(cfblk2) -> cfblk4/1
  cfblk5/1 -> cfblk7/2(cfblk9), cfblk9/2(cfblk8), cfblk6/4(cfblk16)
  cfblk1/1 -> cfblk13/1, cfblk8/4(cfblk11), cfblk5/2
  cfblk8/2(cfblk13) -> cfblk5/1
  cfblk11/1 -> cfblk7/3(cfblk10)
  cfblk9/3(cfblk11) -> cfblk3/1
  cfblk12/1 -> cfblk6/3(cfblk15)
  cfblk6/1(cfblk2) -> cfblk9/1(cfblk1)
  cfblk6/2(cfblk17) -> cfblk18/1, cfblk19/1
  cfblk7/1(cfblk2) -> cfblk14/1
  cfblk14/1 -> cfblk8/2(cfblk9)
  cfblk9/2(cfblk10) -> cfblk15/1
  cfblk15/1 -> cfblk6/2(cfblk14)
  cfblk16/1 -> cfblk8/1(cfblk1)
  cfblk17/1 -> cfblk9/3(cfblk9)
  cfblk18/1 -> cfblk8/3(cfblk10)
  cfblk19/1 -> cfblk8/5(cfblk12)

== system sampleModel20/cfblk84/cfblk6 ==
  cfblk1 : Inport
  cfblk7 : Inport  Port=2
  cfblk8 : Inport  Port=3
  cfblk{11..14} (4 alike) : Delay  SampleTime=1
  cfblk3 : Sqrt  Operator=rSqrt  AlgorithmType=Newton-Raphson  SaturateOnIntegerOverflow=on
  cfblk4 : Subsystem
  cfblk5 : Subsystem
  cfblk6 : Subsystem
  cfblk2 : Outport
  cfblk9 : Outport  Port=2
  cfblk10 : Outport  Port=3
  wires:
  cfblk8/1 -> cfblk5/1(cfblk1), cfblk5/3(cfblk12)
  cfblk3/1 -> cfblk6/1(cfblk1), cfblk6/8(cfblk13)
  cfblk4/1(cfblk2) -> cfblk3/1
  cfblk5/1(cfblk2) -> cfblk11/1, cfblk12/1
  cfblk7/1 -> cfblk6/3(cfblk8), cfblk5/4(cfblk13), cfblk6/6(cfblk11)
  cfblk1/1 -> cfblk10/1, cfblk4/3(cfblk7), cfblk6/4(cfblk9), cfblk6/5(cfblk10), cfblk6/7(cfblk12)
  cfblk6/1(cfblk2) -> cfblk2/1
  cfblk6/2(cfblk15) -> cfblk5/2(cfblk11)
  cfblk6/3(cfblk16) -> cfblk9/1, cfblk13/1, cfblk14/1
  cfblk11/1 -> cfblk6/2(cfblk7)
  cfblk12/1 -> cfblk6/9(cfblk14)
  cfblk13/1 -> cfblk4/1(cfblk1)
  cfblk14/1 -> cfblk4/2(cfblk6)

== system sampleModel20/cfblk84/cfblk7 ==
  cfblk1 : Inport
  cfblk11 : Inport  Port=2
  cfblk12 : Inport  Port=3
  cfblk13 : Inport  Port=4
  cfblk14 : Inport  Port=5
  cfblk15 : Inport  Port=6
  cfblk16 : Inport  Port=7
  cfblk10 : Subsystem
  cfblk{18..21} (4 alike) : Delay  SampleTime=1
  cfblk3 : Sum  Inputs=|++
  cfblk4 : Sum  Inputs=|++
  cfblk5 : Sqrt  Operator=rSqrt  AlgorithmType=Newton-Raphson  SaturateOnIntegerOverflow=on
  cfblk6 : Sum
  cfblk7 : Product  Inputs=**
  cfblk8 : DotProduct  InputSameDT=on  OutDataTypeStr=Inherit: Inherit via internal rule
  cfblk9 : Subsystem
  cfblk2 : Outport
  cfblk17 : Outport  Port=2
  wires:
  cfblk12/1 -> cfblk7/1
  cfblk3/1 -> cfblk7/2, cfblk10/6(cfblk14)
  cfblk11/1 -> cfblk9/1(cfblk1), cfblk10/5(cfblk13)
  cfblk4/1 -> cfblk17/1
  cfblk13/1 -> cfblk10/1(cfblk1)
  cfblk8/1 -> cfblk3/1
  cfblk16/1 -> cfblk2/1
  cfblk10/1(cfblk2) -> cfblk9/2(cfblk8)
  cfblk5/1 -> cfblk6/1, cfblk21/1
  cfblk1/1 -> cfblk8/2
  cfblk14/1 -> cfblk6/2
  cfblk6/1 -> cfblk4/1
  cfblk15/1 -> cfblk10/2(cfblk10)
  cfblk9/2(cfblk13) -> cfblk4/2
  cfblk10/2(cfblk15) -> cfblk9/3(cfblk9)
  cfblk10/3(cfblk16) -> cfblk5/1
  cfblk10/4(cfblk17) -> cfblk9/4(cfblk10), cfblk9/5(cfblk11), cfblk9/6(cfblk12)
  cfblk7/1 -> cfblk18/1
  cfblk18/1 -> cfblk8/1
  cfblk9/1(cfblk2) -> cfblk19/1
  cfblk19/1 -> cfblk3/2
  cfblk9/3(cfblk14) -> cfblk20/1
  cfblk20/1 -> cfblk10/3(cfblk11)
  cfblk21/1 -> cfblk10/4(cfblk12)

== system sampleModel20/cfblk84/cfblk8 ==
  cfblk1 : Inport
  cfblk10 : Inport  Port=2
  cfblk11 : Inport  Port=3
  cfblk12 : Inport  Port=4
  cfblk13 : Inport  Port=5
  cfblk3 : Signum
  cfblk4 : ComplexToMagnitudeAngle
  cfblk5 : Sqrt  SaturateOnIntegerOverflow=on
  cfblk6 : PermuteDimensions
  cfblk7 : Subsystem
  cfblk8 : Subsystem
  cfblk9 : Subsystem
  cfblk2 : Outport
  wires:
  cfblk8/1(cfblk2) -> cfblk5/1
  cfblk12/1 -> cfblk8/1(cfblk1)
  cfblk7/1(cfblk2) -> cfblk8/2(cfblk11)
  cfblk1/1 -> cfblk4/1
  cfblk7/2(cfblk15) -> cfblk6/1
  cfblk10/1 -> cfblk7/1(cfblk1)
  cfblk11/1 -> cfblk7/2(cfblk14)
  cfblk4/1 -> cfblk2/1
  cfblk13/1 -> cfblk3/1
  cfblk6/1 -> cfblk9/1(cfblk1)
  cfblk5/1 -> cfblk9/2(cfblk7)
  cfblk7/3(cfblk16) -> cfblk9/3(cfblk8)
  cfblk3/1 -> cfblk9/4(cfblk9)

== system sampleModel20/cfblk84/cfblk9 ==
  cfblk1 : Inport
  cfblk8 : Inport  Port=2
  cfblk9 : Inport  Port=3
  cfblk{12..15} (4 alike) : Delay  SampleTime=1
  cfblk3 : Sum  Inputs=+
  cfblk4 : Sqrt  Operator=rSqrt  AlgorithmType=Newton-Raphson  SaturateOnIntegerOverflow=on
  cfblk5 : Subsystem
  cfblk6 : Subsystem
  cfblk7 : Subsystem
  cfblk2 : Outport
  cfblk10 : Outport  Port=2
  cfblk11 : Outport  Port=3
  wires:
  cfblk1/1 -> cfblk7/1(cfblk1), cfblk6/7(cfblk14)
  cfblk8/1 -> cfblk4/1, cfblk6/2(cfblk9), cfblk10/1, cfblk6/5(cfblk12)
  cfblk9/1 -> cfblk5/1(cfblk1), cfblk7/2(cfblk9), cfblk6/8(cfblk15)
  cfblk7/1(cfblk2) -> cfblk2/1, cfblk6/3(cfblk10), cfblk5/4(cfblk11)
  cfblk5/1(cfblk2) -> cfblk11/1, cfblk13/1
  cfblk6/1(cfblk2) -> cfblk3/1
  cfblk6/2(cfblk16) -> cfblk5/2(cfblk9), cfblk14/1, cfblk15/1
  cfblk4/1 -> cfblk5/3(cfblk10), cfblk6/4(cfblk11), cfblk7/5(cfblk12)
  cfblk3/1 -> cfblk12/1
  cfblk12/1 -> cfblk6/1(cfblk1)
  cfblk13/1 -> cfblk6/6(cfblk13)
  cfblk14/1 -> cfblk7/3(cfblk10)
  cfblk15/1 -> cfblk7/4(cfblk11)

== system sampleModel20/cfblk85/cfblk10 ==
  cfblk1 : Inport
  cfblk7 : Inport  Port=2
  cfblk8 : Inport  Port=3
  cfblk9 : Inport  Port=4
  cfblk10 : Inport  Port=5
  cfblk11 : Inport  Port=6
  cfblk12 : Delay  SampleTime=1
  cfblk3 : Product  Inputs=*
  cfblk4 : MinMax
  cfblk5 : Gain  Gain=[861925874.669645]
  cfblk6 : Subsystem
  cfblk2 : Outport
  wires:
  cfblk7/1 -> cfblk2/1
  cfblk11/1 -> cfblk3/1, cfblk6/7(cfblk12)
  cfblk1/1 -> cfblk4/1
  cfblk4/1 -> cfblk6/1(cfblk1)
  cfblk6/1(cfblk2) -> cfblk5/1
  cfblk9/1 -> cfblk6/3(cfblk8)
  cfblk10/1 -> cfblk6/4(cfblk9)
  cfblk3/1 -> cfblk6/5(cfblk10)
  cfblk8/1 -> cfblk6/6(cfblk11)
  cfblk5/1 -> cfblk12/1
  cfblk12/1 -> cfblk6/2(cfblk7)

== system sampleModel20/cfblk85/cfblk9 ==
  cfblk1 : Inport
  cfblk10 : Inport  Port=2
  cfblk11 : Inport  Port=3
  cfblk12 : Inport  Port=4
  cfblk{13..19} (7 alike) : Delay  SampleTime=1
  cfblk3 : Sqrt  SaturateOnIntegerOverflow=on
  cfblk4 : Product
  cfblk5 : UnaryMinus
  cfblk6 : Subsystem
  cfblk7 : Subsystem
  cfblk8 : Subsystem
  cfblk9 : Subsystem
  cfblk2 : Outport
  wires:
  cfblk12/1 -> cfblk2/1, cfblk8/3(cfblk11)
  cfblk5/1 -> cfblk4/2, cfblk13/1, cfblk17/1
  cfblk4/1 -> cfblk7/1(cfblk1), cfblk15/1, cfblk16/1
  cfblk1/1 -> cfblk8/2(cfblk10)
  cfblk10/1 -> cfblk4/1
  cfblk8/1(cfblk2) -> cfblk6/2(cfblk6)
  cfblk11/1 -> cfblk6/3(cfblk7)
  cfblk9/1(cfblk2) -> cfblk5/1
  cfblk6/1(cfblk2) -> cfblk9/2(cfblk11)
  cfblk6/2(cfblk10) -> cfblk9/3(cfblk12)
  cfblk9/2(cfblk13) -> cfblk3/1, cfblk18/1
  cfblk13/1 -> cfblk6/1(cfblk1)
  cfblk7/1(cfblk2) -> cfblk14/1
  cfblk14/1 -> cfblk8/1(cfblk1)
  cfblk15/1 -> cfblk6/5(cfblk9)
  cfblk16/1 -> cfblk8/4(cfblk12)
  cfblk17/1 -> cfblk8/5(cfblk13)
  cfblk18/1 -> cfblk6/4(cfblk8)
  cfblk3/1 -> cfblk19/1
  cfblk19/1 -> cfblk9/1(cfblk1)

== system sampleModel20/cfblk86/cfblk8 ==
  cfblk1 : Inport
  cfblk4 : Inport  Port=2
  cfblk5 : Inport  Port=3
  cfblk6 : Inport  Port=4
  cfblk7 : Inport  Port=5
  cfblk3 : Subsystem
  cfblk2 : Outport
  wires:
  cfblk3/1(cfblk2) -> cfblk2/1
  cfblk6/1 -> cfblk3/1(cfblk1)
  cfblk7/1 -> cfblk3/2(cfblk14)
  cfblk4/1 -> cfblk3/3(cfblk15)

== system sampleModel20/cfblk86/cfblk9 ==
  cfblk1 : Inport
  cfblk11 : Inport  Port=2
  cfblk12 : Inport  Port=3
  cfblk13 : Inport  Port=4
  cfblk14 : Inport  Port=5
  cfblk15 : Inport  Port=6
  cfblk10 : Subsystem
  cfblk{17..21} (5 alike) : Delay  SampleTime=1
  cfblk3 : Sum  Inputs=+
  cfblk4 : Subsystem
  cfblk5 : Subsystem
  cfblk6 : Subsystem
  cfblk7 : Subsystem
  cfblk8 : Subsystem
  cfblk9 : Subsystem
  cfblk2 : Outport
  cfblk16 : Outport  Port=2
  wires:
  cfblk8/1(cfblk2) -> cfblk10/1(cfblk1)
  cfblk1/1 -> cfblk7/1(cfblk1), cfblk8/8(cfblk14)
  cfblk11/1 -> cfblk8/1(cfblk1), cfblk5/3(cfblk14), cfblk4/3(cfblk14)
  cfblk9/2(cfblk14) -> cfblk16/1
  cfblk3/1 -> cfblk9/1(cfblk1), cfblk8/6(cfblk12)
  cfblk7/1(cfblk2) -> cfblk2/1
  cfblk4/1(cfblk2) -> cfblk5/1(cfblk1)
  cfblk6/1(cfblk2) -> cfblk5/2(cfblk13)
  cfblk4/2(cfblk15) -> cfblk7/2(cfblk9)
  cfblk14/1 -> cfblk3/1
  cfblk12/1 -> cfblk9/2(cfblk11), cfblk6/2(cfblk9)
  cfblk13/1 -> cfblk8/3(cfblk9)
  cfblk9/3(cfblk15) -> cfblk5/4(cfblk15), cfblk20/1
  cfblk15/1 -> cfblk4/1(cfblk1), cfblk9/4(cfblk13)
  cfblk4/3(cfblk16) -> cfblk6/1(cfblk1)
  cfblk10/2(cfblk9) -> cfblk4/2(cfblk13), cfblk9/3(cfblk12), cfblk21/1
  cfblk10/1(cfblk2) -> cfblk17/1
  cfblk17/1 -> cfblk8/2(cfblk8)
  cfblk5/1(cfblk2) -> cfblk18/1
  cfblk18/1 -> cfblk8/4(cfblk10)
  cfblk9/1(cfblk2) -> cfblk19/1
  cfblk19/1 -> cfblk10/2(cfblk8)
  cfblk20/1 -> cfblk8/5(cfblk11)
  cfblk21/1 -> cfblk8/7(cfblk13)

== system sampleModel20/cfblk87/cfblk5 ==
  cfblk1 : Inport
  cfblk12 : Inport  Port=2
  cfblk13 : Inport  Port=3
  cfblk14 : Inport  Port=4
  cfblk15 : Inport  Port=5
  cfblk10 : Subsystem
  cfblk11 : Subsystem
  cfblk{16..24} (9 alike) : Delay  SampleTime=1
  cfblk3 : Product
  cfblk4 : Sum  Inputs=+-
  cfblk5 : Assignment  DiagnosticForDimensions=Warning  IndexOptions=Index vector (dialog)  Indices=1  OutputSizes=1
  cfblk6 : Math  Operator=conj  SaturateOnIntegerOverflow=on
  cfblk7 : Subsystem
  cfblk8 : Subsystem
  cfblk9 : Subsystem
  cfblk2 : Outport
  wires:
  cfblk4/1 -> cfblk19/1, cfblk20/1
  cfblk5/1 -> cfblk11/3(cfblk12), cfblk11/6(cfblk15), cfblk17/1, cfblk22/1, cfblk23/1, cfblk24/1
  cfblk9/1(cfblk2) -> cfblk2/1
  cfblk6/1 -> cfblk4/1, cfblk9/9(cfblk14)
  cfblk12/1 -> cfblk11/1(cfblk1), cfblk9/4(cfblk9)
  cfblk14/1 -> cfblk9/1(cfblk1), cfblk7/4(cfblk10), cfblk10/3(cfblk8)
  cfblk13/1 -> cfblk11/2(cfblk11), cfblk10/1(cfblk1), cfblk11/5(cfblk14)
  cfblk8/1(cfblk2) -> cfblk3/1
  cfblk10/1(cfblk2) -> cfblk4/2
  cfblk7/1(cfblk2) -> cfblk8/2(cfblk11)
  cfblk11/1(cfblk2) -> cfblk10/4(cfblk9), cfblk18/1, cfblk21/1
  cfblk7/2(cfblk14) -> cfblk9/2(cfblk7)
  cfblk9/2(cfblk16) -> cfblk5/2, cfblk11/4(cfblk13)
  cfblk15/1 -> cfblk6/1, cfblk8/4(cfblk13), cfblk7/6(cfblk12), cfblk9/10(cfblk15)
  cfblk8/2(cfblk15) -> cfblk9/3(cfblk8), cfblk10/2(cfblk7), cfblk3/2, cfblk11/7(cfblk16), cfblk9/8(cfblk13)
  cfblk1/1 -> cfblk7/2(cfblk8), cfblk7/7(cfblk13), cfblk8/5(cfblk14)
  cfblk3/1 -> cfblk16/1
  cfblk16/1 -> cfblk7/1(cfblk1)
  cfblk17/1 -> cfblk8/1(cfblk1)
  cfblk18/1 -> cfblk8/3(cfblk12)
  cfblk19/1 -> cfblk5/1
  cfblk20/1 -> cfblk9/5(cfblk10)
  cfblk21/1 -> cfblk9/6(cfblk11)
  cfblk22/1 -> cfblk7/3(cfblk9)
  cfblk23/1 -> cfblk7/5(cfblk11)
  cfblk24/1 -> cfblk9/7(cfblk12)

== system sampleModel20/cfblk87/cfblk6 ==
  cfblk1 : Inport
  cfblk13 : Inport  Port=2
  cfblk14 : Inport  Port=3
  cfblk10 : Subsystem
  cfblk11 : Subsystem
  cfblk12 : Subsystem
  cfblk{16..22} (7 alike) : Delay  SampleTime=1
  cfblk3 : DotProduct  InputSameDT=on  OutDataTypeStr=Inherit: Inherit via internal rule
  cfblk4 : Bias  Bias=[-392929766.388138]
  cfblk5 : Polyval  Coefs=[ +2.081618890e-019, -1.441693666e-014, +4.719686976e-010, -8.536869453e-006, +1.621573104e-001, -8.087801117e+001 ]
  cfblk6 : PermuteDimensions
  cfblk7 : Sum  Inputs=+-
  cfblk8 : Sqrt  Operator=rSqrt  AlgorithmType=Newton-Raphson  SaturateOnIntegerOverflow=on
  cfblk9 : Sum  Inputs=+-
  cfblk2 : Outport
  cfblk15 : Outport  Port=2
  wires:
  cfblk12/1(cfblk2) -> cfblk2/1
  cfblk1/1 -> cfblk9/1
  cfblk12/2(cfblk16) -> cfblk9/2
  cfblk9/1 -> cfblk15/1
  cfblk13/1 -> cfblk3/1
  cfblk6/1 -> cfblk10/1(cfblk1)
  cfblk14/1 -> cfblk10/2(cfblk8), cfblk12/4(cfblk14)
  cfblk5/1 -> cfblk7/1, cfblk12/5(cfblk15), cfblk10/4(cfblk10), cfblk22/1
  cfblk4/1 -> cfblk11/1(cfblk1)
  cfblk11/1(cfblk2) -> cfblk6/1
  cfblk8/1 -> cfblk3/2, cfblk16/1, cfblk17/1, cfblk18/1
  cfblk11/3(cfblk12) -> cfblk10/3(cfblk9)
  cfblk3/1 -> cfblk7/2
  cfblk10/1(cfblk2) -> cfblk8/1
  cfblk7/1 -> cfblk12/1(cfblk1), cfblk12/2(cfblk12)
  cfblk10/2(cfblk12) -> cfblk12/3(cfblk13), cfblk19/1, cfblk20/1
  cfblk11/4(cfblk13) -> cfblk5/1
  cfblk16/1 -> cfblk11/3(cfblk7)
  cfblk17/1 -> cfblk11/6(cfblk10)
  cfblk18/1 -> cfblk10/5(cfblk11)
  cfblk19/1 -> cfblk11/2(cfblk6)
  cfblk20/1 -> cfblk11/5(cfblk9)
  cfblk11/2(cfblk11) -> cfblk21/1
  cfblk21/1 -> cfblk4/1
  cfblk22/1 -> cfblk11/4(cfblk8)

== system sampleModel20/cfblk87/cfblk7 ==
  cfblk1 : Inport
  cfblk13 : Inport  Port=2
  cfblk14 : Inport  Port=3
  cfblk15 : Inport  Port=4
  cfblk10 : Subsystem
  cfblk11 : Subsystem
  cfblk12 : Subsystem
  cfblk{16..19} (4 alike) : Delay  SampleTime=1
  cfblk3 : Sqrt  SaturateOnIntegerOverflow=on
  cfblk4 : Sum  Inputs=|++
  cfblk5 : Sum  Inputs=+
  cfblk6 : Math  Operator=conj  SaturateOnIntegerOverflow=on
  cfblk7 : Sin  TimeSource=Use external signal  SampleTime=0
  cfblk8 : ComplexToMagnitudeAngle
  cfblk9 : Subsystem
  cfblk2 : Outport
  wires:
  cfblk13/1 -> cfblk7/1, cfblk11/4(cfblk14)
  cfblk5/1 -> cfblk2/1
  cfblk1/1 -> cfblk6/1
  cfblk10/1(cfblk2) -> cfblk11/1(cfblk1)
  cfblk14/1 -> cfblk11/2(cfblk12)
  cfblk7/1 -> cfblk12/1(cfblk1)
  cfblk12/1(cfblk2) -> cfblk4/1, cfblk8/1
  cfblk6/1 -> cfblk5/1
  cfblk8/1 -> cfblk3/1
  cfblk4/1 -> cfblk11/3(cfblk13)
  cfblk15/1 -> cfblk4/2, cfblk10/3(cfblk14)
  cfblk8/2 -> cfblk9/1(cfblk1), cfblk10/5(cfblk16)
  cfblk11/3(cfblk17) -> cfblk18/1, cfblk19/1
  cfblk3/1 -> cfblk9/4(cfblk14), cfblk11/5(cfblk15)
  cfblk9/1(cfblk2) -> cfblk10/2(cfblk13), cfblk10/4(cfblk15)
  cfblk11/1(cfblk2) -> cfblk16/1
  cfblk16/1 -> cfblk10/1(cfblk1)
  cfblk11/2(cfblk16) -> cfblk17/1
  cfblk17/1 -> cfblk9/2(cfblk12)
  cfblk18/1 -> cfblk9/3(cfblk13)
  cfblk19/1 -> cfblk9/5(cfblk15)

== system sampleModel20/cfblk87/cfblk8 ==
  cfblk1 : Inport
  cfblk8 : Inport  Port=2
  cfblk9 : Inport  Port=3
  cfblk10 : Inport  Port=4
  cfblk11 : Inport  Port=5
  cfblk14 : Delay  SampleTime=1
  cfblk15 : Delay  SampleTime=1
  cfblk3 : Sqrt  SaturateOnIntegerOverflow=on
  cfblk4 : Signum
  cfblk5 : Sin  TimeSource=Use external signal  SampleTime=0
  cfblk6 : Subsystem
  cfblk7 : Subsystem
  cfblk2 : Outport
  cfblk12 : Outport  Port=2
  cfblk13 : Outport  Port=3
  wires:
  cfblk6/1(cfblk2) -> cfblk12/1
  cfblk6/2(cfblk17) -> cfblk5/1
  cfblk1/1 -> cfblk6/1(cfblk1)
  cfblk11/1 -> cfblk3/1
  cfblk10/1 -> cfblk4/1
  cfblk3/1 -> cfblk7/1(cfblk1), cfblk7/5(cfblk7)
  cfblk8/1 -> cfblk7/2(cfblk4), cfblk6/3(cfblk15)
  cfblk5/1 -> cfblk7/3(cfblk5)
  cfblk4/1 -> cfblk2/1
  cfblk9/1 -> cfblk7/4(cfblk6)
  cfblk7/1(cfblk2) -> cfblk13/1
  cfblk7/2(cfblk8) -> cfblk14/1, cfblk15/1
  cfblk14/1 -> cfblk6/2(cfblk14)
  cfblk15/1 -> cfblk6/4(cfblk16)

== system sampleModel20/cfblk87/cfblk9 ==
  cfblk1 : Inport
  cfblk9 : Inport  Port=2
  cfblk10 : Inport  Port=3
  cfblk11 : Inport  Port=4
  cfblk12 : Inport  Port=5
  cfblk13 : Inport  Port=6
  cfblk16 : Delay  SampleTime=1
  cfblk17 : Delay  SampleTime=1
  cfblk3 : Reshape
  cfblk4 : Bias  Bias=[944880885.809281]
  cfblk5 : Subsystem
  cfblk6 : Subsystem
  cfblk7 : Subsystem
  cfblk8 : Subsystem
  cfblk2 : Outport
  cfblk14 : Outport  Port=2
  cfblk15 : Outport  Port=3
  wires:
  cfblk1/1 -> cfblk5/1(cfblk1)
  cfblk6/1(cfblk2) -> cfblk14/1
  cfblk9/1 -> cfblk8/1(cfblk1)
  cfblk4/1 -> cfblk2/1
  cfblk5/1(cfblk2) -> cfblk7/1(cfblk1)
  cfblk10/1 -> cfblk7/2(cfblk5)
  cfblk12/1 -> cfblk7/3(cfblk6), cfblk8/5(cfblk9)
  cfblk8/1(cfblk2) -> cfblk3/1
  cfblk3/1 -> cfblk15/1
  cfblk7/1(cfblk2) -> cfblk4/1
  cfblk13/1 -> cfblk6/1(cfblk1), cfblk8/3(cfblk7)
  cfblk11/1 -> cfblk5/3(cfblk15)
  cfblk8/4(cfblk12) -> cfblk6/2(cfblk10)
  cfblk7/2(cfblk8) -> cfblk8/2(cfblk6)
  cfblk7/3(cfblk9) -> cfblk6/3(cfblk11), cfblk8/4(cfblk8)
  cfblk8/2(cfblk10) -> cfblk16/1
  cfblk16/1 -> cfblk7/4(cfblk7)
  cfblk8/3(cfblk11) -> cfblk17/1
  cfblk17/1 -> cfblk5/2(cfblk14)

== system sampleModel20/cfblk88/cfblk5 ==
  cfblk1 : Inport
  cfblk9 : Inport  Port=2
  cfblk{10..13} (4 alike) : Delay  SampleTime=1
  cfblk3 : Abs
  cfblk4 : UnaryMinus
  cfblk5 : Bias  Bias=[754714598.980117]
  cfblk6 : Subsystem
  cfblk7 : Subsystem
  cfblk8 : Subsystem
  cfblk2 : Outport
  wires:
  cfblk6/1(cfblk2) -> cfblk7/1(cfblk1), cfblk8/2(cfblk13), cfblk8/3(cfblk14)
  cfblk1/1 -> cfblk3/1, cfblk7/2(cfblk6)
  cfblk8/1(cfblk2) -> cfblk4/1, cfblk13/1
  cfblk3/1 -> cfblk6/1(cfblk1)
  cfblk4/1 -> cfblk7/3(cfblk7), cfblk12/1
  cfblk9/1 -> cfblk8/1(cfblk1)
  cfblk7/1(cfblk2) -> cfblk5/1
  cfblk5/1 -> cfblk2/1
  cfblk7/2(cfblk8) -> cfblk10/1, cfblk11/1
  cfblk10/1 -> cfblk6/3(cfblk11)
  cfblk11/1 -> cfblk6/4(cfblk12)
  cfblk12/1 -> cfblk6/2(cfblk10)
  cfblk13/1 -> cfblk6/5(cfblk13)

== system sampleModel20/cfblk88/cfblk6 ==
  cfblk1 : Inport
  cfblk10 : Inport  Port=2
  cfblk11 : Inport  Port=3
  cfblk12 : Inport  Port=4
  cfblk13 : Inport  Port=5
  cfblk14 : Inport  Port=6
  cfblk15 : Inport  Port=7
  cfblk16 : Inport  Port=8
  cfblk18 : Delay  SampleTime=1
  cfblk3 : Sum
  cfblk4 : Product
  cfblk5 : MinMax  Inputs=3
  cfblk6 : Subsystem
  cfblk7 : Subsystem
  cfblk8 : Subsystem
  cfblk9 : Subsystem
  cfblk2 : Outport
  cfblk17 : Outport  Port=2
  wires:
  cfblk13/1 -> cfblk6/1(cfblk1)
  cfblk5/1 -> cfblk17/1
  cfblk6/1(cfblk2) -> cfblk4/1
  cfblk7/1(cfblk2) -> cfblk9/1(cfblk1)
  cfblk16/1 -> cfblk4/2
  cfblk9/1(cfblk2) -> cfblk3/1
  cfblk10/1 -> cfblk7/1(cfblk1)
  cfblk15/1 -> cfblk9/2(cfblk5), cfblk5/3
  cfblk11/1 -> cfblk3/2
  cfblk7/2(cfblk10) -> cfblk2/1
  cfblk9/2(cfblk7) -> cfblk8/1(cfblk1)
  cfblk14/1 -> cfblk8/2(cfblk8)
  cfblk12/1 -> cfblk6/2(cfblk7)
  cfblk6/2(cfblk8) -> cfblk8/3(cfblk9)
  cfblk4/1 -> cfblk7/2(cfblk9)
  cfblk3/1 -> cfblk5/1
  cfblk1/1 -> cfblk5/2
  cfblk8/1(cfblk2) -> cfblk18/1
  cfblk18/1 -> cfblk9/3(cfblk6)

== system sampleModel20/cfblk89/cfblk7 ==
  cfblk1 : Inport
  cfblk7 : Inport  Port=2
  cfblk8 : Inport  Port=3
  cfblk10 : Delay  SampleTime=1
  cfblk3 : Bias  Bias=[-848621423.457961]
  cfblk4 : Polyval  Coefs=[ +2.081618890e-019, -1.441693666e-014, +4.719686976e-010, -8.536869453e-006, +1.621573104e-001, -8.087801117e+001 ]
  cfblk5 : Trigonometry
  cfblk6 : Subsystem
  cfblk2 : Outport
  cfblk9 : Outport  Port=2
  wires:
  cfblk7/1 -> cfblk2/1
  cfblk8/1 -> cfblk6/1(cfblk1)
  cfblk5/1 -> cfblk3/1
  cfblk4/1 -> cfblk9/1
  cfblk1/1 -> cfblk6/3(cfblk12), cfblk6/4(cfblk13)
  cfblk6/1(cfblk2) -> cfblk5/1
  cfblk6/2(cfblk14) -> cfblk4/1
  cfblk3/1 -> cfblk10/1
  cfblk10/1 -> cfblk6/2(cfblk11)

== system sampleModel20/cfblk89/cfblk8 ==
  cfblk1 : Inport
  cfblk10 : Inport  Port=2
  cfblk{11..17} (7 alike) : Delay  SampleTime=1
  cfblk3 : Sum  Inputs=+-
  cfblk4 : Sum  Inputs=+
  cfblk5 : Gain  Gain=[275607793.395297]
  cfblk6 : Subsystem
  cfblk7 : Subsystem
  cfblk8 : Subsystem
  cfblk9 : Subsystem
  cfblk2 : Outport
  wires:
  cfblk8/1(cfblk2) -> cfblk9/1(cfblk1)
  cfblk5/1 -> cfblk2/1, cfblk12/1, cfblk13/1, cfblk14/1
  cfblk10/1 -> cfblk3/1, cfblk7/4(cfblk15)
  cfblk9/1(cfblk2) -> cfblk7/1(cfblk1)
  cfblk6/1(cfblk2) -> cfblk3/2
  cfblk9/2(cfblk13) -> cfblk7/2(cfblk13), cfblk17/1
  cfblk3/1 -> cfblk4/1
  cfblk7/2(cfblk16) -> cfblk5/1, cfblk15/1, cfblk16/1
  cfblk1/1 -> cfblk6/1(cfblk1)
  cfblk4/1 -> cfblk8/2(cfblk11), cfblk8/4(cfblk13)
  cfblk7/1(cfblk2) -> cfblk11/1
  cfblk11/1 -> cfblk9/2(cfblk12)
  cfblk12/1 -> cfblk7/3(cfblk14)
  cfblk13/1 -> cfblk6/3(cfblk15)
  cfblk14/1 -> cfblk6/4(cfblk16)
  cfblk15/1 -> cfblk8/3(cfblk12)
  cfblk16/1 -> cfblk6/2(cfblk14)
  cfblk17/1 -> cfblk8/1(cfblk1)

== system sampleModel20/cfblk89/cfblk9 ==
  cfblk1 : Inport
  cfblk9 : Inport  Port=2
  cfblk10 : Inport  Port=3
  cfblk11 : Inport  Port=4
  cfblk12 : Inport  Port=5
  cfblk14 : Delay  SampleTime=1
  cfblk15 : Delay  SampleTime=1
  cfblk16 : Delay  SampleTime=1
  cfblk3 : Sum  Inputs=+-
  cfblk4 : Math  Operator=transpose  SaturateOnIntegerOverflow=on
  cfblk5 : Subsystem
  cfblk6 : Subsystem
  cfblk7 : Subsystem
  cfblk8 : Subsystem
  cfblk2 : Outport
  cfblk13 : Outport  Port=2
  wires:
  cfblk1/1 -> cfblk5/1(cfblk1)
  cfblk12/1 -> cfblk6/1(cfblk1), cfblk6/5(cfblk10)
  cfblk10/1 -> cfblk3/1, cfblk7/4(cfblk11)
  cfblk6/1(cfblk2) -> cfblk3/2
  cfblk4/1 -> cfblk13/1
  cfblk3/1 -> cfblk8/1(cfblk1)
  cfblk6/2(cfblk11) -> cfblk8/2(cfblk12)
  cfblk8/1(cfblk2) -> cfblk2/1
  cfblk7/1(cfblk2) -> cfblk8/3(cfblk13)
  cfblk9/1 -> cfblk4/1
  cfblk11/1 -> cfblk6/2(cfblk7), cfblk7/3(cfblk10)
  cfblk5/1(cfblk2) -> cfblk6/3(cfblk8)
  cfblk5/2(cfblk16) -> cfblk6/4(cfblk9), cfblk7/2(cfblk9)
  cfblk6/4(cfblk13) -> cfblk7/1(cfblk1)
  cfblk8/2(cfblk14) -> cfblk14/1
  cfblk14/1 -> cfblk5/3(cfblk14)
  cfblk6/3(cfblk12) -> cfblk15/1
  cfblk15/1 -> cfblk5/4(cfblk15)
  cfblk7/2(cfblk12) -> cfblk16/1
  cfblk16/1 -> cfblk5/2(cfblk13)

== system sampleModel20/cfblk90/cfblk8 ==
  cfblk1 : Inport
  cfblk6 : Inport  Port=2
  cfblk7 : Inport  Port=3
  cfblk8 : Inport  Port=4
  cfblk9 : Inport  Port=5
  cfblk10 : Inport  Port=6
  cfblk12 : Delay  SampleTime=1
  cfblk3 : simulink/Math Operations/MinMax Running Resettable  Function=min  vinit=0.0
  cfblk4 : Bias  Bias=[-517635864.512233]
  cfblk5 : Subsystem
  cfblk2 : Outport
  cfblk11 : Outport  Port=2
  wires:
  cfblk7/1 -> cfblk2/1
  cfblk8/1 -> cfblk5/1(cfblk1)
  cfblk6/1 -> cfblk11/1
  cfblk10/1 -> cfblk3/1
  cfblk1/1 -> cfblk5/3(cfblk8)
  cfblk5/1(cfblk2) -> cfblk3/2
  cfblk5/2(cfblk9) -> cfblk4/1
  cfblk4/1 -> cfblk12/1
  cfblk12/1 -> cfblk5/2(cfblk7)

== system sampleModel20/cfblk90/cfblk9 ==
  cfblk1 : Inport
  cfblk11 : Inport  Port=2
  cfblk12 : Inport  Port=3
  cfblk13 : Inport  Port=4
  cfblk14 : Inport  Port=5
  cfblk15 : Inport  Port=6
  cfblk10 : Subsystem
  cfblk{18..21} (4 alike) : Delay  SampleTime=1
  cfblk3 : Sum  Inputs=+
  cfblk4 : Assignment  DiagnosticForDimensions=Warning  IndexOptions=Index vector (dialog)  Indices=1  OutputSizes=1
  cfblk5 : Rounding
  cfblk6 : Subsystem
  cfblk7 : Subsystem
  cfblk8 : Subsystem
  cfblk9 : Subsystem
  cfblk2 : Outport
  cfblk16 : Outport  Port=2
  cfblk17 : Outport  Port=3
  wires:
  cfblk13/1 -> cfblk10/1(cfblk1)
  cfblk6/1(cfblk2) -> cfblk3/1
  cfblk11/1 -> cfblk16/1
  cfblk8/1(cfblk2) -> cfblk4/1
  cfblk6/2(cfblk12) -> cfblk17/1
  cfblk10/1(cfblk2) -> cfblk8/1(cfblk1)
  cfblk3/1 -> cfblk5/1
  cfblk12/1 -> cfblk8/2(cfblk5)
  cfblk5/1 -> cfblk4/2
  cfblk14/1 -> cfblk6/1(cfblk1)
  cfblk8/2(cfblk7) -> cfblk6/2(cfblk10)
  cfblk10/2(cfblk11) -> cfblk8/3(cfblk6)
  cfblk9/1(cfblk2) -> cfblk6/3(cfblk11)
  cfblk1/1 -> cfblk7/5(cfblk14)
  cfblk7/1(cfblk2) -> cfblk2/1
  cfblk15/1 -> cfblk9/1(cfblk1)
  cfblk7/2(cfblk15) -> cfblk9/2(cfblk11)
  cfblk7/3(cfblk16) -> cfblk9/3(cfblk12)
  cfblk4/1 -> cfblk18/1
  cfblk18/1 -> cfblk7/1(cfblk1)
  cfblk6/3(cfblk13) -> cfblk19/1
  cfblk19/1 -> cfblk7/2(cfblk11)
  cfblk9/2(cfblk13) -> cfblk20/1
  cfblk20/1 -> cfblk7/3(cfblk12)
  cfblk9/3(cfblk14) -> cfblk21/1
  cfblk21/1 -> cfblk7/4(cfblk13)

== system sampleModel20/cfblk91/cfblk5 ==
  cfblk1 : Inport
  cfblk11 : Inport  Port=2
  cfblk10 : Subsystem
  cfblk{12..23} (12 alike) : Delay  SampleTime=1
  cfblk3 : PermuteDimensions
  cfblk4 : Subsystem
  cfblk5 : Subsystem
  cfblk6 : Subsystem
  cfblk7 : Subsystem
  cfblk8 : Subsystem
  cfblk9 : Subsystem
  cfblk2 : Outport
  wires:
  cfblk6/1(cfblk2) -> cfblk2/1
  cfblk4/1(cfblk2) -> cfblk8/1(cfblk1)
  cfblk9/2(cfblk16) -> cfblk10/3(cfblk15), cfblk15/1, cfblk16/1, cfblk20/1, cfblk21/1
  cfblk1/1 -> cfblk7/2(cfblk9), cfblk9/2(cfblk13), cfblk10/4(cfblk16)
  cfblk8/1(cfblk2) -> cfblk3/1
  cfblk11/1 -> cfblk8/2(cfblk9)
  cfblk3/1 -> cfblk6/2(cfblk6), cfblk9/4(cfblk15), cfblk12/1, cfblk13/1
  cfblk5/1(cfblk2) -> cfblk4/2(cfblk6)
  cfblk10/1(cfblk2) -> cfblk17/1, cfblk18/1, cfblk19/1
  cfblk7/1(cfblk2) -> cfblk5/3(cfblk11)
  cfblk6/2(cfblk7) -> cfblk9/1(cfblk1), cfblk10/2(cfblk14), cfblk22/1
  cfblk7/2(cfblk13) -> cfblk6/1(cfblk1)
  cfblk7/3(cfblk14) -> cfblk10/1(cfblk1), cfblk9/3(cfblk14)
  cfblk12/1 -> cfblk4/1(cfblk1)
  cfblk13/1 -> cfblk7/5(cfblk12)
  cfblk9/1(cfblk2) -> cfblk14/1
  cfblk14/1 -> cfblk7/1(cfblk1)
  cfblk15/1 -> cfblk5/1(cfblk1)
  cfblk16/1 -> cfblk5/4(cfblk12)
  cfblk17/1 -> cfblk7/3(cfblk10)
  cfblk18/1 -> cfblk7/4(cfblk11)
  cfblk19/1 -> cfblk4/3(cfblk7)
  cfblk20/1 -> cfblk8/3(cfblk10)
  cfblk21/1 -> cfblk8/4(cfblk11)
  cfblk22/1 -> cfblk5/5(cfblk13)
  cfblk8/2(cfblk12) -> cfblk23/1
  cfblk23/1 -> cfblk5/2(cfblk10)

== system sampleModel20/cfblk91/cfblk6 ==
  cfblk1 : Inport
  cfblk7 : Inport  Port=2
  cfblk8 : Inport  Port=3
  cfblk9 : Inport  Port=4
  cfblk12 : Delay  SampleTime=1
  cfblk3 : UnaryMinus
  cfblk4 : Sin  TimeSource=Use external signal  SampleTime=0
  cfblk5 : Assignment  DiagnosticForDimensions=Warning  IndexOptions=Index vector (dialog)  Indices=1  OutputSizes=1
  cfblk6 : Sum  Inputs=|++
  cfblk2 : Outport
  cfblk10 : Outport  Port=2
  cfblk11 : Outport  Port=3
  wires:
  cfblk5/1 -> cfblk2/1
  cfblk1/1 -> cfblk11/1
  cfblk3/1 -> cfblk10/1
  cfblk7/1 -> cfblk3/1, cfblk6/2
  cfblk8/1 -> cfblk5/1
  cfblk9/1 -> cfblk5/2
  cfblk4/1 -> cfblk6/1
  cfblk6/1 -> cfblk12/1
  cfblk12/1 -> cfblk4/1

== system sampleModel20/cfblk91/cfblk7 ==
  cfblk1 : Inport
  cfblk6 : Inport  Port=2
  cfblk7 : Inport  Port=3
  cfblk3 : Squeeze
  cfblk4 : Subsystem
  cfblk5 : Subsystem
  cfblk2 : Outport
  cfblk8 : Outport  Port=2
  wires:
  cfblk4/1(cfblk2) -> cfblk8/1
  cfblk7/1 -> cfblk5/1(cfblk1)
  cfblk6/1 -> cfblk5/2(cfblk6), cfblk4/3(cfblk6)
  cfblk1/1 -> cfblk3/1, cfblk4/4(cfblk7), cfblk4/7(cfblk10), cfblk4/9(cfblk12)
  cfblk3/1 -> cfblk4/1(cfblk1), cfblk4/5(cfblk8)
  cfblk5/1(cfblk2) -> cfblk2/1
  cfblk5/2(cfblk7) -> cfblk4/2(cfblk5), cfblk4/6(cfblk9), cfblk4/8(cfblk11)
